simulink model "mod_simple2_oxygen"  (R2014a)
settings: Solver=ode45  StartTime=0.0  StopTime=10.0  RelTol=1e-3
settings Model: Creator=Tanay  LastModifiedBy=Tanay

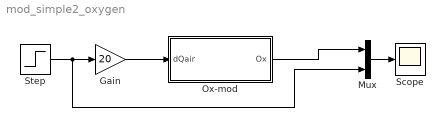
== system mod_simple2_oxygen ==
  Gain : Gain  Gain=20
  Mux : Mux  Inputs=2
  Ox-mod : Subsystem  mask{cx_max=10, alpha=1, beta=1}
      mask prompts: cx_max "Oxygen contents"; alpha "Liquefication speed"; beta "Aeration coef."
  Scope : Scope
  Step : Step  SampleTime=0
  wires:
  Ox-mod/1(Ox) -> Mux/1
  Step/1 -> Mux/2, Gain/1
  Gain/1 -> Ox-mod/1(dQair)
  Mux/1 -> Scope/1

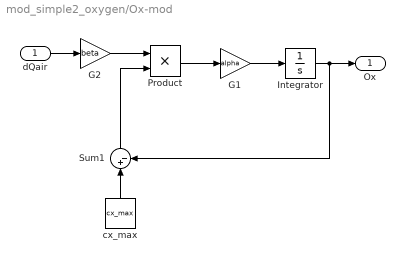
== system mod_simple2_oxygen/Ox-mod ==
  dQair : Inport
  G1 : Gain  Gain=alpha
  G2 : Gain  Gain=beta
  Integrator : Integrator
  Product : Product
  Sum1 : Sum  Inputs=|+-
  cx_max : Constant  Value=cx_max
  Ox : Outport
  wires:
  Sum1/1 -> Product/2
  cx_max/1 -> Sum1/1
  dQair/1 -> G2/1
  Product/1 -> G1/1
  Integrator/1 -> Sum1/2, Ox/1
  G1/1 -> Integrator/1
  G2/1 -> Product/1
